simulink model "bh_6dof_NEWTON_vs_LAGRANGE"  (R2020b)
settings: Solver=ode23t  StartTime=0.0  StopTime=200  FixedStep=0.001  RelTol=1e-5  EnableMultiTasking=on
undefined symbols (not defined in the file or in its folder): P_elec, P_mot, P_one_prop, P_rot, P_veh, P_veh_no_props, sigbuilder_block
libraries: bh_6dof_LIBRARY x45, simulink_extras x37, pid_lib x24, simulink x6
(part 5 of 5)

== system bh_6dof_NEWTON_vs_LAGRANGE/PLANT VEHICLE_SYS1/bh_6DOF (Euler Angles, Lagrangian, Multi_body)/integrate/create_st_BUS ==
  e : Inport
  x : Inport  Port=2
  e_dot : Inport  Port=3
  x_dot : Inport  Port=4
  Bus Creator : BusCreator  Inputs=4
  Bus Creator1 : BusCreator  Inputs=6
  Bus Creator2 : BusCreator  Inputs=6
  Demux{,1..3} (4 alike) : Demux  Outputs=3
  Mux : Mux  Inputs=2
  Mux1 : Mux  Inputs=2
  Reshape1 : Reshape  OutputDimensionality=Column vector (2-D)
  Reshape8 : Reshape  OutputDimensionality=Column vector (2-D)
  state_BUS : Outport  VectorParamsAs1DForOutWhenUnconnected=off
  wires:
  e/1 -> Mux/1, [e]
  x/1 -> Mux/2, [x]
  e_dot/1 -> Mux1/1, [eD]
  x_dot/1 -> Mux1/2, [xD]
  Mux1/1 -> Reshape1/1
  Mux/1 -> Reshape8/1
  Reshape1/1 -> Bus Creator/2  "vel_col"
  Reshape8/1 -> Bus Creator/1  "pos_col"
  Bus Creator1/1 -> Bus Creator/3  "Pos_list"
  Demux/1 -> Bus Creator1/1  "Phi"
  Demux/2 -> Bus Creator1/2  "Theta"
  Demux/3 -> Bus Creator1/3  "Psi"
  Demux1/2 -> Bus Creator1/5  "Y"
  Demux1/3 -> Bus Creator1/6  "Z"
  Demux1/1 -> Bus Creator1/4  "X"
  [e] -> Demux/1
  [x] -> Demux1/1
  Bus Creator2/1 -> Bus Creator/4  "Vel_list"
  Demux2/1 -> Bus Creator2/1  "Phi_D"
  Demux2/2 -> Bus Creator2/2  "Theta_D"
  Demux2/3 -> Bus Creator2/3  "Psi_D"
  Demux3/1 -> Bus Creator2/4  "X_D"
  Demux3/2 -> Bus Creator2/5  "Y_D"
  Demux3/3 -> Bus Creator2/6  "Z_D"
  [eD] -> Demux2/1
  [xD] -> Demux3/1
  Bus Creator/1 -> state_BUS/1

== matlab function bh_6dof_NEWTON_vs_LAGRANGE/PLANT VEHICLE_SYS1/bh_6DOF (Euler Angles, Lagrangian, Multi_body)/MATLAB Function1 ==
  data: I input; Ixx output; Ixy output; Ixz output; Iyy output; Iyz output; Izz output
function [Ixx, Ixy, Ixz, Iyy, Iyz, Izz] = fcn(I)

Ixx = I(1,1); 
Ixy = I(1,2); 
Ixz = I(1,3); 
Iyy = I(2,2); 
Iyz = I(2,3); 
Izz = I(3,3);

end

== matlab function bh_6dof_NEWTON_vs_LAGRANGE/PLANT VEHICLE_SYS1/bh_6DOF (Euler Angles, Lagrangian, Multi_body)/MATLAB Function ==
  data: I input; Ixx output; Ixy output; Ixz output; Iyy output; Iyz output; Izz output
function [Ixx, Ixy, Ixz, Iyy, Iyz, Izz] = fcn(I)

Ixx = I(1,1); 
Ixy = I(1,2); 
Ixz = I(1,3); 
Iyy = I(2,2); 
Iyz = I(2,3); 
Izz = I(3,3);

end

== matlab function bh_6dof_NEWTON_vs_LAGRANGE/PLANT VEHICLE_SYS1/bh_6DOF (Euler Angles, Lagrangian, Multi_body)/Vg_to_Vb/bRg1 ==
  data: phi input; bRg output; theta input; psi input
function bRg = bRg(phi,theta,psi)
%#codegen

%    This function was generated by the Symbolic Math Toolbox version 7.2.
%    28-Aug-2017 09:46:25

bRg = reshape([cos(phi).*cos(theta),-cos(psi).*sin(phi)+cos(phi).*sin(psi).*sin(theta),sin(phi).*sin(psi)+cos(phi).*cos(psi).*sin(theta),cos(theta).*sin(phi),cos(phi).*cos(psi)+sin(phi).*sin(psi).*sin(theta),-cos(phi).*sin(psi)+cos(psi).*sin(phi).*sin(theta),-sin(theta),cos(theta).*sin(psi),cos(psi).*cos(theta)],[3,3]);

== matlab function bh_6dof_NEWTON_vs_LAGRANGE/PLANT VEHICLE_SYS1/bh_6DOF (Euler Angles, Lagrangian, Multi_body)/bRg ==
  data: phi input; bRg output; theta input; psi input
function bRg = bRg(phi,theta,psi)
%#codegen

%    This function was generated by the Symbolic Math Toolbox version 7.2.
%    28-Aug-2017 08:55:21

bRg = reshape([cos(phi).*cos(theta),-cos(psi).*sin(phi)+cos(phi).*sin(psi).*sin(theta),sin(phi).*sin(psi)+cos(phi).*cos(psi).*sin(theta),cos(theta).*sin(phi),cos(phi).*cos(psi)+sin(phi).*sin(psi).*sin(theta),-cos(phi).*sin(psi)+cos(psi).*sin(phi).*sin(theta),-sin(theta),cos(theta).*sin(psi),cos(psi).*cos(theta)],[3,3]);

== matlab function bh_6dof_NEWTON_vs_LAGRANGE/PLANT VEHICLE_SYS1/bh_6DOF (Euler Angles, Lagrangian, Multi_body)/MCKGQ1 ==
  data: I_xx input; M output; I_xy input; I_xz input; I_yy input; I_yz input; I_zz input; Iprop_xx input; Iprop_xy input; Iprop_xz input; Iprop_yy input; Iprop_yz input; Iprop_zz input; Mbz_1 input; Mbz_2 input; Mbz_3 input; Mbz_4 input; THE_Phi input; THE_Psi input; THE_Phi_D input; THE_Psi_D input; THE_Theta input; THE_Theta_D input; Tbz_1 input; Tbz_2 input; Tbz_3 input; Tbz_4 input; cg_to_mot_H input; cg_to_mot_L input; g input; m input; mprop input; wMOT_1 input; wMOT_2 input; wMOT_3 input; wMOT_4 input; C output; K output; G output; Q output
function [M,C,K,G,Q] = MCKGQ(I_xx,I_xy,I_xz,I_yy,I_yz,I_zz,Iprop_xx,Iprop_xy,Iprop_xz,Iprop_yy,Iprop_yz,Iprop_zz,Mbz_1,Mbz_2,Mbz_3,Mbz_4,THE_Phi,THE_Psi,THE_Phi_D,THE_Psi_D,THE_Theta,THE_Theta_D,Tbz_1,Tbz_2,Tbz_3,Tbz_4,cg_to_mot_H,cg_to_mot_L,g,m,mprop,wMOT_1,wMOT_2,wMOT_3,wMOT_4)
%#codegen

%    This function was generated by the Symbolic Math Toolbox version 7.2.
%    07-Sep-2017 08:25:18

M = reshape([I_xx+Iprop_xx.*4.0+cg_to_mot_H.^2.*mprop.*4.0+cg_to_mot_L.^2.*mprop.*2.0-I_xx.*cos(THE_Theta).^2+I_yy.*cos(THE_Theta).^2-Iprop_xx.*cos(THE_Theta).^2.*4.0+Iprop_yy.*cos(THE_Theta).^2.*4.0-I_yy.*cos(THE_Psi).^2.*cos(THE_Theta).^2+I_zz.*cos(THE_Psi).^2.*cos(THE_Theta).^2-Iprop_yy.*cos(THE_Psi).^2.*cos(THE_Theta).^2.*4.0+Iprop_zz.*cos(THE_Psi).^2.*cos(THE_Theta).^2.*4.0+I_yz.*cos(THE_Psi).*cos(THE_Theta).^2.*sin(THE_Psi).*2.0+Iprop_yz.*cos(THE_Psi).*cos(THE_Theta).^2.*sin(THE_Psi).*8.0-cg_to_mot_H.^2.*mprop.*cos(THE_Psi).^2.*cos(THE_Theta).^2.*4.0+cg_to_mot_L.^2.*mprop.*cos(THE_Psi).^2.*cos(THE_Theta).^2.*2.0-I_xz.*cos(THE_Psi).*cos(THE_Theta).*sin(THE_Theta).*2.0-Iprop_xz.*cos(THE_Psi).*cos(THE_Theta).*sin(THE_Theta).*8.0-I_xy.*cos(THE_Theta).*sin(THE_Psi).*sin(THE_Theta).*2.0-Iprop_xy.*cos(THE_Theta).*sin(THE_Psi).*sin(THE_Theta).*8.0,-I_yz.*cos(THE_Theta)-Iprop_yz.*cos(THE_Theta).*4.0-I_xy.*cos(THE_Psi).*sin(THE_Theta)-Iprop_xy.*cos(THE_Psi).*sin(THE_Theta).*4.0+I_xz.*sin(THE_Psi).*sin(THE_Theta)+Iprop_xz.*sin(THE_Psi).*sin(THE_Theta).*4.0+I_yz.*cos(THE_Psi).^2.*cos(THE_Theta).*2.0+Iprop_yz.*cos(THE_Psi).^2.*cos(THE_Theta).*8.0+I_yy.*cos(THE_Psi).*cos(THE_Theta).*sin(THE_Psi)-I_zz.*cos(THE_Psi).*cos(THE_Theta).*sin(THE_Psi)+Iprop_yy.*cos(THE_Psi).*cos(THE_Theta).*sin(THE_Psi).*4.0-Iprop_zz.*cos(THE_Psi).*cos(THE_Theta).*sin(THE_Psi).*4.0+cg_to_mot_H.^2.*mprop.*cos(THE_Psi).*cos(THE_Theta).*sin(THE_Psi).*4.0-cg_to_mot_L.^2.*mprop.*cos(THE_Psi).*cos(THE_Theta).*sin(THE_Psi).*2.0,-I_xx.*sin(THE_Theta)-Iprop_xx.*sin(THE_Theta).*4.0+I_xz.*cos(THE_Psi).*cos(THE_Theta)+Iprop_xz.*cos(THE_Psi).*cos(THE_Theta).*4.0+I_xy.*cos(THE_Theta).*sin(THE_Psi)+Iprop_xy.*cos(THE_Theta).*sin(THE_Psi).*4.0-cg_to_mot_H.^2.*mprop.*sin(THE_Theta).*4.0-cg_to_mot_L.^2.*mprop.*sin(THE_Theta).*2.0,cg_to_mot_H.*mprop.*(cos(THE_Phi).*sin(THE_Psi)-cos(THE_Psi).*sin(THE_Phi).*sin(THE_Theta)).*4.0,cg_to_mot_H.*mprop.*(sin(THE_Phi).*sin(THE_Psi)+cos(THE_Phi).*cos(THE_Psi).*sin(THE_Theta)).*4.0,0.0,-I_yz.*cos(THE_Theta)-Iprop_yz.*cos(THE_Theta).*4.0-I_xy.*cos(THE_Psi).*sin(THE_Theta)-Iprop_xy.*cos(THE_Psi).*sin(THE_Theta).*4.0+I_xz.*sin(THE_Psi).*sin(THE_Theta)+Iprop_xz.*sin(THE_Psi).*sin(THE_Theta).*4.0+I_yz.*cos(THE_Psi).^2.*cos(THE_Theta).*2.0+Iprop_yz.*cos(THE_Psi).^2.*cos(THE_Theta).*8.0+I_yy.*cos(THE_Psi).*cos(THE_Theta).*sin(THE_Psi)-I_zz.*cos(THE_Psi).*cos(THE_Theta).*sin(THE_Psi)+Iprop_yy.*cos(THE_Psi).*cos(THE_Theta).*sin(THE_Psi).*4.0-Iprop_zz.*cos(THE_Psi).*cos(THE_Theta).*sin(THE_Psi).*4.0+cg_to_mot_H.^2.*mprop.*cos(THE_Psi).*cos(THE_Theta).*sin(THE_Psi).*4.0-cg_to_mot_L.^2.*mprop.*cos(THE_Psi).*cos(THE_Theta).*sin(THE_Psi).*2.0,I_zz+Iprop_zz.*4.0+cg_to_mot_L.^2.*mprop.*4.0+I_yy.*cos(THE_Psi).^2-I_zz.*cos(THE_Psi).^2+Iprop_yy.*cos(THE_Psi).^2.*4.0-Iprop_zz.*cos(THE_Psi).^2.*4.0-I_yz.*sin(THE_Psi.*2.0)-Iprop_yz.*sin(THE_Psi.*2.0).*4.0+cg_to_mot_H.^2.*mprop.*cos(THE_Psi).^2.*4.0-cg_to_mot_L.^2.*mprop.*cos(THE_Psi).^2.*2.0,I_xy.*cos(THE_Psi)+Iprop_xy.*cos(THE_Psi).*4.0-I_xz.*sin(THE_Psi)-Iprop_xz.*sin(THE_Psi).*4.0,cg_to_mot_H.*mprop.*cos(THE_Phi).*cos(THE_Psi).*cos(THE_Theta).*4.0,cg_to_mot_H.*mprop.*cos(THE_Psi).*cos(THE_Theta).*sin(THE_Phi).*4.0,cg_to_mot_H.*mprop.*cos(THE_Psi).*sin(THE_Theta).*-4.0,-I_xx.*sin(THE_Theta)-Iprop_xx.*sin(THE_Theta).*4.0+I_xz.*cos(THE_Psi).*cos(THE_Theta)+Iprop_xz.*cos(THE_Psi).*cos(THE_Theta).*4.0+I_xy.*cos(THE_Theta).*sin(THE_Psi)+Iprop_xy.*cos(THE_Theta).*sin(THE_Psi).*4.0-cg_to_mot_H.^2.*mprop.*sin(THE_Theta).*4.0-cg_to_mot_L.^2.*mprop.*sin(THE_Theta).*2.0,I_xy.*cos(THE_Psi)+Iprop_xy.*cos(THE_Psi).*4.0-I_xz.*sin(THE_Psi)-Iprop_xz.*sin(THE_Psi).*4.0,I_xx+Iprop_xx.*4.0+cg_to_mot_H.^2.*mprop.*4.0+cg_to_mot_L.^2.*mprop.*2.0,cg_to_mot_H.*mprop.*(cos(THE_Psi).*sin(THE_Phi)-cos(THE_Phi).*sin(THE_Psi).*sin(THE_Theta)).*4.0,cg_to_mot_H.*mprop.*(cos(THE_Phi).*cos(THE_Psi)+sin(THE_Phi).*sin(THE_Psi).*sin(THE_Theta)).*-4.0,cg_to_mot_H.*mprop.*cos(THE_Theta).*sin(THE_Psi).*-4.0,cg_to_mot_H.*mprop.*(cos(THE_Phi).*sin(THE_Psi)-cos(THE_Psi).*sin(THE_Phi).*sin(THE_Theta)).*4.0,cg_to_mot_H.*mprop.*cos(THE_Phi).*cos(THE_Psi).*cos(THE_Theta).*4.0,cg_to_mot_H.*mprop.*(cos(THE_Psi).*sin(THE_Phi)-cos(THE_Phi).*sin(THE_Psi).*sin(THE_Theta)).*4.0,m+mprop.*4.0,0.0,0.0,cg_to_mot_H.*mprop.*(sin(THE_Phi).*sin(THE_Psi)+cos(THE_Phi).*cos(THE_Psi).*sin(THE_Theta)).*4.0,cg_to_mot_H.*mprop.*cos(THE_Psi).*cos(THE_Theta).*sin(THE_Phi).*4.0,cg_to_mot_H.*mprop.*(cos(THE_Phi).*cos(THE_Psi)+sin(THE_Phi).*sin(THE_Psi).*sin(THE_Theta)).*-4.0,0.0,m+mprop.*4.0,0.0,0.0,cg_to_mot_H.*mprop.*cos(THE_Psi).*sin(THE_Theta).*-4.0,cg_to_mot_H.*mprop.*cos(THE_Theta).*sin(THE_Psi).*-4.0,0.0,0.0,m+mprop.*4.0],[6,6]);
if nargout > 1
    C = reshape([I_yz.*THE_Psi_D.*cos(THE_Theta).^2.*-2.0-Iprop_yz.*THE_Psi_D.*cos(THE_Theta).^2.*8.0+I_xx.*THE_Theta_D.*sin(THE_Theta.*2.0)-I_yy.*THE_Theta_D.*sin(THE_Theta.*2.0)+Iprop_xx.*THE_Theta_D.*sin(THE_Theta.*2.0).*4.0-Iprop_yy.*THE_Theta_D.*sin(THE_Theta.*2.0).*4.0+I_xz.*THE_Theta_D.*cos(THE_Psi).*2.0+Iprop_xz.*THE_Theta_D.*cos(THE_Psi).*8.0+I_xy.*THE_Theta_D.*sin(THE_Psi).*2.0+Iprop_xy.*THE_Theta_D.*sin(THE_Psi).*8.0+I_yz.*THE_Psi_D.*cos(THE_Psi).^2.*cos(THE_Theta).^2.*4.0+Iprop_yz.*THE_Psi_D.*cos(THE_Psi).^2.*cos(THE_Theta).^2.*1.6e1-I_xz.*THE_Theta_D.*cos(THE_Psi).*cos(THE_Theta).^2.*4.0-Iprop_xz.*THE_Theta_D.*cos(THE_Psi).*cos(THE_Theta).^2.*1.6e1-I_xy.*THE_Theta_D.*cos(THE_Theta).^2.*sin(THE_Psi).*4.0-Iprop_xy.*THE_Theta_D.*cos(THE_Theta).^2.*sin(THE_Psi).*1.6e1-I_xy.*THE_Psi_D.*cos(THE_Psi).*cos(THE_Theta).*sin(THE_Theta).*2.0-Iprop_xy.*THE_Psi_D.*cos(THE_Psi).*cos(THE_Theta).*sin(THE_Theta).*8.0+I_xz.*THE_Psi_D.*cos(THE_Theta).*sin(THE_Psi).*sin(THE_Theta).*2.0+Iprop_xz.*THE_Psi_D.*cos(THE_Theta).*sin(THE_Psi).*sin(THE_Theta).*8.0+I_yy.*THE_Psi_D.*cos(THE_Psi).*cos(THE_Theta).^2.*sin(THE_Psi).*2.0-I_zz.*THE_Psi_D.*cos(THE_Psi).*cos(THE_Theta).^2.*sin(THE_Psi).*2.0+I_yy.*THE_Theta_D.*cos(THE_Psi).^2.*cos(THE_Theta).*sin(THE_Theta).*2.0-I_zz.*THE_Theta_D.*cos(THE_Psi).^2.*cos(THE_Theta).*sin(THE_Theta).*2.0+Iprop_yy.*THE_Psi_D.*cos(THE_Psi).*cos(THE_Theta).^2.*sin(THE_Psi).*8.0-Iprop_zz.*THE_Psi_D.*cos(THE_Psi).*cos(THE_Theta).^2.*sin(THE_Psi).*8.0+Iprop_yy.*THE_Theta_D.*cos(THE_Psi).^2.*cos(THE_Theta).*sin(THE_Theta).*8.0-Iprop_zz.*THE_Theta_D.*cos(THE_Psi).^2.*cos(THE_Theta).*sin(THE_Theta).*8.0+THE_Psi_D.*cg_to_mot_H.^2.*mprop.*cos(THE_Psi).*cos(THE_Theta).^2.*sin(THE_Psi).*8.0-THE_Psi_D.*cg_to_mot_L.^2.*mprop.*cos(THE_Psi).*cos(THE_Theta).^2.*sin(THE_Psi).*4.0+THE_Theta_D.*cg_to_mot_H.^2.*mprop.*cos(THE_Psi).^2.*cos(THE_Theta).*sin(THE_Theta).*8.0-THE_Theta_D.*cg_to_mot_L.^2.*mprop.*cos(THE_Psi).^2.*cos(THE_Theta).*sin(THE_Theta).*4.0-I_yz.*THE_Theta_D.*cos(THE_Psi).*cos(THE_Theta).*sin(THE_Psi).*sin(THE_Theta).*4.0-Iprop_yz.*THE_Theta_D.*cos(THE_Psi).*cos(THE_Theta).*sin(THE_Psi).*sin(THE_Theta).*1.6e1,I_xx.*THE_Phi_D.*sin(THE_Theta.*2.0).*(-1.0./2.0)+I_yy.*THE_Phi_D.*sin(THE_Theta.*2.0).*(1.0./2.0)-Iprop_xx.*THE_Phi_D.*sin(THE_Theta.*2.0).*2.0+Iprop_yy.*THE_Phi_D.*sin(THE_Theta.*2.0).*2.0-I_xz.*THE_Phi_D.*cos(THE_Psi)+I_xx.*THE_Psi_D.*cos(THE_Theta)-I_yy.*THE_Psi_D.*cos(THE_Theta)+I_zz.*THE_Psi_D.*cos(THE_Theta)-Iprop_xz.*THE_Phi_D.*cos(THE_Psi).*4.0+Iprop_xx.*THE_Psi_D.*cos(THE_Theta).*4.0-Iprop_yy.*THE_Psi_D.*cos(THE_Theta).*4.0+Iprop_zz.*THE_Psi_D.*cos(THE_Theta).*4.0-I_xy.*THE_Phi_D.*sin(THE_Psi)-Iprop_xy.*THE_Phi_D.*sin(THE_Psi).*4.0+Iprop_xz.*wMOT_1.*cos(THE_Theta)+Iprop_xz.*wMOT_2.*cos(THE_Theta)+Iprop_xz.*wMOT_3.*cos(THE_Theta)+Iprop_xz.*wMOT_4.*cos(THE_Theta)+I_xz.*THE_Psi_D.*cos(THE_Psi).*sin(THE_Theta).*2.0+Iprop_xz.*THE_Psi_D.*cos(THE_Psi).*sin(THE_Theta).*8.0+I_xy.*THE_Psi_D.*sin(THE_Psi).*sin(THE_Theta).*2.0+Iprop_xy.*THE_Psi_D.*sin(THE_Psi).*sin(THE_Theta).*8.0+THE_Psi_D.*cg_to_mot_L.^2.*mprop.*cos(THE_Theta).*4.0+Iprop_zz.*wMOT_1.*cos(THE_Psi).*sin(THE_Theta)+Iprop_zz.*wMOT_2.*cos(THE_Psi).*sin(THE_Theta)+Iprop_zz.*wMOT_3.*cos(THE_Psi).*sin(THE_Theta)+Iprop_zz.*wMOT_4.*cos(THE_Psi).*sin(THE_Theta)+Iprop_yz.*wMOT_1.*sin(THE_Psi).*sin(THE_Theta)+Iprop_yz.*wMOT_2.*sin(THE_Psi).*sin(THE_Theta)+Iprop_yz.*wMOT_3.*sin(THE_Psi).*sin(THE_Theta)+Iprop_yz.*wMOT_4.*sin(THE_Psi).*sin(THE_Theta)+I_xz.*THE_Phi_D.*cos(THE_Psi).*cos(THE_Theta).^2.*2.0+I_yy.*THE_Psi_D.*cos(THE_Psi).^2.*cos(THE_Theta).*2.0-I_zz.*THE_Psi_D.*cos(THE_Psi).^2.*cos(THE_Theta).*2.0+Iprop_xz.*THE_Phi_D.*cos(THE_Psi).*cos(THE_Theta).^2.*8.0+Iprop_yy.*THE_Psi_D.*cos(THE_Psi).^2.*cos(THE_Theta).*8.0-Iprop_zz.*THE_Psi_D.*cos(THE_Psi).^2.*cos(THE_Theta).*8.0+I_xy.*THE_Phi_D.*cos(THE_Theta).^2.*sin(THE_Psi).*2.0+Iprop_xy.*THE_Phi_D.*cos(THE_Theta).^2.*sin(THE_Psi).*8.0-I_yz.*THE_Psi_D.*cos(THE_Psi).*cos(THE_Theta).*sin(THE_Psi).*4.0-Iprop_yz.*THE_Psi_D.*cos(THE_Psi).*cos(THE_Theta).*sin(THE_Psi).*1.6e1-I_yy.*THE_Phi_D.*cos(THE_Psi).^2.*cos(THE_Theta).*sin(THE_Theta)+I_zz.*THE_Phi_D.*cos(THE_Psi).^2.*cos(THE_Theta).*sin(THE_Theta)-Iprop_yy.*THE_Phi_D.*cos(THE_Psi).^2.*cos(THE_Theta).*sin(THE_Theta).*4.0+Iprop_zz.*THE_Phi_D.*cos(THE_Psi).^2.*cos(THE_Theta).*sin(THE_Theta).*4.0+THE_Psi_D.*cg_to_mot_H.^2.*mprop.*cos(THE_Psi).^2.*cos(THE_Theta).*8.0-THE_Psi_D.*cg_to_mot_L.^2.*mprop.*cos(THE_Psi).^2.*cos(THE_Theta).*4.0-THE_Phi_D.*cg_to_mot_H.^2.*mprop.*cos(THE_Psi).^2.*cos(THE_Theta).*sin(THE_Theta).*4.0+THE_Phi_D.*cg_to_mot_L.^2.*mprop.*cos(THE_Psi).^2.*cos(THE_Theta).*sin(THE_Theta).*2.0+I_yz.*THE_Phi_D.*cos(THE_Psi).*cos(THE_Theta).*sin(THE_Psi).*sin(THE_Theta).*2.0+Iprop_yz.*THE_Phi_D.*cos(THE_Psi).*cos(THE_Theta).*sin(THE_Psi).*sin(THE_Theta).*8.0,I_yz.*THE_Phi_D.*cos(THE_Theta).^2+Iprop_yz.*THE_Phi_D.*cos(THE_Theta).^2.*4.0-I_xx.*THE_Theta_D.*cos(THE_Theta)+I_yy.*THE_Theta_D.*cos(THE_Theta)-I_zz.*THE_Theta_D.*cos(THE_Theta)-Iprop_xx.*THE_Theta_D.*cos(THE_Theta).*4.0+Iprop_yy.*THE_Theta_D.*cos(THE_Theta).*4.0-Iprop_zz.*THE_Theta_D.*cos(THE_Theta).*4.0-I_yz.*THE_Phi_D.*cos(THE_Psi).^2.*cos(THE_Theta).^2.*2.0-Iprop_yz.*THE_Phi_D.*cos(THE_Psi).^2.*cos(THE_Theta).^2.*8.0-I_xz.*THE_Theta_D.*cos(THE_Psi).*sin(THE_Theta).*2.0-Iprop_xz.*THE_Theta_D.*cos(THE_Psi).*sin(THE_Theta).*8.0-I_xy.*THE_Theta_D.*sin(THE_Psi).*sin(THE_Theta).*2.0-Iprop_xy.*THE_Theta_D.*sin(THE_Psi).*sin(THE_Theta).*8.0-Iprop_yz.*wMOT_1.*cos(THE_Psi).*cos(THE_Theta)-Iprop_yz.*wMOT_2.*cos(THE_Psi).*cos(THE_Theta)-Iprop_yz.*wMOT_3.*cos(THE_Psi).*cos(THE_Theta)-Iprop_yz.*wMOT_4.*cos(THE_Psi).*cos(THE_Theta)-THE_Theta_D.*cg_to_mot_L.^2.*mprop.*cos(THE_Theta).*4.0+Iprop_zz.*wMOT_1.*cos(THE_Theta).*sin(THE_Psi)+Iprop_zz.*wMOT_2.*cos(THE_Theta).*sin(THE_Psi)+Iprop_zz.*wMOT_3.*cos(THE_Theta).*sin(THE_Psi)+Iprop_zz.*wMOT_4.*cos(THE_Theta).*sin(THE_Psi)-I_yy.*THE_Theta_D.*cos(THE_Psi).^2.*cos(THE_Theta).*2.0+I_zz.*THE_Theta_D.*cos(THE_Psi).^2.*cos(THE_Theta).*2.0-Iprop_yy.*THE_Theta_D.*cos(THE_Psi).^2.*cos(THE_Theta).*8.0+Iprop_zz.*THE_Theta_D.*cos(THE_Psi).^2.*cos(THE_Theta).*8.0+I_xy.*THE_Phi_D.*cos(THE_Psi).*cos(THE_Theta).*sin(THE_Theta)+I_yz.*THE_Theta_D.*cos(THE_Psi).*cos(THE_Theta).*sin(THE_Psi).*4.0+Iprop_xy.*THE_Phi_D.*cos(THE_Psi).*cos(THE_Theta).*sin(THE_Theta).*4.0+Iprop_yz.*THE_Theta_D.*cos(THE_Psi).*cos(THE_Theta).*sin(THE_Psi).*1.6e1-I_xz.*THE_Phi_D.*cos(THE_Theta).*sin(THE_Psi).*sin(THE_Theta)-Iprop_xz.*THE_Phi_D.*cos(THE_Theta).*sin(THE_Psi).*sin(THE_Theta).*4.0-I_yy.*THE_Phi_D.*cos(THE_Psi).*cos(THE_Theta).^2.*sin(THE_Psi)+I_zz.*THE_Phi_D.*cos(THE_Psi).*cos(THE_Theta).^2.*sin(THE_Psi)-Iprop_yy.*THE_Phi_D.*cos(THE_Psi).*cos(THE_Theta).^2.*sin(THE_Psi).*4.0+Iprop_zz.*THE_Phi_D.*cos(THE_Psi).*cos(THE_Theta).^2.*sin(THE_Psi).*4.0-THE_Theta_D.*cg_to_mot_H.^2.*mprop.*cos(THE_Psi).^2.*cos(THE_Theta).*8.0+THE_Theta_D.*cg_to_mot_L.^2.*mprop.*cos(THE_Psi).^2.*cos(THE_Theta).*4.0-THE_Phi_D.*cg_to_mot_H.^2.*mprop.*cos(THE_Psi).*cos(THE_Theta).^2.*sin(THE_Psi).*4.0+THE_Phi_D.*cg_to_mot_L.^2.*mprop.*cos(THE_Psi).*cos(THE_Theta).^2.*sin(THE_Psi).*2.0,cg_to_mot_H.*mprop.*(THE_Psi_D.*cos(THE_Phi).*cos(THE_Psi).*-2.0+THE_Phi_D.*sin(THE_Phi).*sin(THE_Psi)-THE_Psi_D.*sin(THE_Phi).*sin(THE_Psi).*sin(THE_Theta).*2.0+THE_Phi_D.*cos(THE_Phi).*cos(THE_Psi).*sin(THE_Theta)+THE_Theta_D.*cos(THE_Psi).*cos(THE_Theta).*sin(THE_Phi).*2.0).*-4.0,cg_to_mot_H.*mprop.*(THE_Phi_D.*cos(THE_Phi).*sin(THE_Psi)+THE_Psi_D.*cos(THE_Psi).*sin(THE_Phi).*2.0+THE_Theta_D.*cos(THE_Phi).*cos(THE_Psi).*cos(THE_Theta).*2.0-THE_Phi_D.*cos(THE_Psi).*sin(THE_Phi).*sin(THE_Theta)-THE_Psi_D.*cos(THE_Phi).*sin(THE_Psi).*sin(THE_Theta).*2.0).*4.0,0.0,-I_xx.*THE_Psi_D.*cos(THE_Theta)-I_yy.*THE_Psi_D.*cos(THE_Theta)+I_zz.*THE_Psi_D.*cos(THE_Theta)-Iprop_xx.*THE_Psi_D.*cos(THE_Theta).*4.0-Iprop_yy.*THE_Psi_D.*cos(THE_Theta).*4.0+Iprop_zz.*THE_Psi_D.*cos(THE_Theta).*4.0+I_yz.*THE_Theta_D.*sin(THE_Theta)+Iprop_yz.*THE_Theta_D.*sin(THE_Theta).*4.0-Iprop_xz.*wMOT_1.*cos(THE_Theta)-Iprop_xz.*wMOT_2.*cos(THE_Theta)-Iprop_xz.*wMOT_3.*cos(THE_Theta)-Iprop_xz.*wMOT_4.*cos(THE_Theta)-I_xy.*THE_Theta_D.*cos(THE_Psi).*cos(THE_Theta)-Iprop_xy.*THE_Theta_D.*cos(THE_Psi).*cos(THE_Theta).*4.0+I_xz.*THE_Theta_D.*cos(THE_Theta).*sin(THE_Psi)+Iprop_xz.*THE_Theta_D.*cos(THE_Theta).*sin(THE_Psi).*4.0-THE_Psi_D.*cg_to_mot_H.^2.*mprop.*cos(THE_Theta).*8.0-Iprop_zz.*wMOT_1.*cos(THE_Psi).*sin(THE_Theta)-Iprop_zz.*wMOT_2.*cos(THE_Psi).*sin(THE_Theta)-Iprop_zz.*wMOT_3.*cos(THE_Psi).*sin(THE_Theta)-Iprop_zz.*wMOT_4.*cos(THE_Psi).*sin(THE_Theta)-Iprop_yz.*wMOT_1.*sin(THE_Psi).*sin(THE_Theta)-Iprop_yz.*wMOT_2.*sin(THE_Psi).*sin(THE_Theta)-Iprop_yz.*wMOT_3.*sin(THE_Psi).*sin(THE_Theta)-Iprop_yz.*wMOT_4.*sin(THE_Psi).*sin(THE_Theta)+I_yy.*THE_Psi_D.*cos(THE_Psi).^2.*cos(THE_Theta).*2.0-I_zz.*THE_Psi_D.*cos(THE_Psi).^2.*cos(THE_Theta).*2.0+Iprop_yy.*THE_Psi_D.*cos(THE_Psi).^2.*cos(THE_Theta).*8.0-Iprop_zz.*THE_Psi_D.*cos(THE_Psi).^2.*cos(THE_Theta).*8.0-I_yz.*THE_Theta_D.*cos(THE_Psi).^2.*sin(THE_Theta).*2.0-Iprop_yz.*THE_Theta_D.*cos(THE_Psi).^2.*sin(THE_Theta).*8.0-I_yz.*THE_Psi_D.*cos(THE_Psi).*cos(THE_Theta).*sin(THE_Psi).*4.0-Iprop_yz.*THE_Psi_D.*cos(THE_Psi).*cos(THE_Theta).*sin(THE_Psi).*1.6e1-I_yy.*THE_Theta_D.*cos(THE_Psi).*sin(THE_Psi).*sin(THE_Theta)+I_zz.*THE_Theta_D.*cos(THE_Psi).*sin(THE_Psi).*sin(THE_Theta)-Iprop_yy.*THE_Theta_D.*cos(THE_Psi).*sin(THE_Psi).*sin(THE_Theta).*4.0+Iprop_zz.*THE_Theta_D.*cos(THE_Psi).*sin(THE_Psi).*sin(THE_Theta).*4.0+THE_Psi_D.*cg_to_mot_H.^2.*mprop.*cos(THE_Psi).^2.*cos(THE_Theta).*8.0-THE_Psi_D.*cg_to_mot_L.^2.*mprop.*cos(THE_Psi).^2.*cos(THE_Theta).*4.0-THE_Theta_D.*cg_to_mot_H.^2.*mprop.*cos(THE_Psi).*sin(THE_Psi).*sin(THE_Theta).*4.0+THE_Theta_D.*cg_to_mot_L.^2.*mprop.*cos(THE_Psi).*sin(THE_Psi).*sin(THE_Theta).*2.0,-THE_Psi_D.*(I_yz.*cos(THE_Psi.*2.0).*2.0+Iprop_yz.*cos(THE_Psi.*2.0).*8.0+I_yy.*sin(THE_Psi.*2.0)-I_zz.*sin(THE_Psi.*2.0)+Iprop_yy.*sin(THE_Psi.*2.0).*4.0-Iprop_zz.*sin(THE_Psi.*2.0).*4.0+cg_to_mot_H.^2.*mprop.*sin(THE_Psi.*2.0).*4.0-cg_to_mot_L.^2.*mprop.*sin(THE_Psi.*2.0).*2.0),I_yz.*THE_Theta_D.*cos(THE_Psi.*2.0)+Iprop_yz.*THE_Theta_D.*cos(THE_Psi.*2.0).*4.0+I_yy.*THE_Theta_D.*sin(THE_Psi.*2.0).*(1.0./2.0)-I_zz.*THE_Theta_D.*sin(THE_Psi.*2.0).*(1.0./2.0)+Iprop_yy.*THE_Theta_D.*sin(THE_Psi.*2.0).*2.0-Iprop_zz.*THE_Theta_D.*sin(THE_Psi.*2.0).*2.0+Iprop_zz.*wMOT_1.*cos(THE_Psi)+Iprop_zz.*wMOT_2.*cos(THE_Psi)+Iprop_zz.*wMOT_3.*cos(THE_Psi)+Iprop_zz.*wMOT_4.*cos(THE_Psi)+Iprop_yz.*wMOT_1.*sin(THE_Psi)+Iprop_yz.*wMOT_2.*sin(THE_Psi)+Iprop_yz.*wMOT_3.*sin(THE_Psi)+Iprop_yz.*wMOT_4.*sin(THE_Psi)+THE_Theta_D.*cg_to_mot_H.^2.*mprop.*sin(THE_Psi.*2.0).*2.0-THE_Theta_D.*cg_to_mot_L.^2.*mprop.*sin(THE_Psi.*2.0),cg_to_mot_H.*mprop.*cos(THE_Phi).*(THE_Psi_D.*cos(THE_Theta).*sin(THE_Psi).*2.0+THE_Theta_D.*cos(THE_Psi).*sin(THE_Theta)).*-4.0,cg_to_mot_H.*mprop.*sin(THE_Phi).*(THE_Psi_D.*cos(THE_Theta).*sin(THE_Psi).*2.0+THE_Theta_D.*cos(THE_Psi).*sin(THE_Theta)).*-4.0,cg_to_mot_H.*mprop.*(THE_Theta_D.*cos(THE_Psi).*cos(THE_Theta)-THE_Psi_D.*sin(THE_Psi).*sin(THE_Theta).*2.0).*-4.0,cos(THE_Theta).*(I_xy.*THE_Psi_D.*cos(THE_Psi)+Iprop_xy.*THE_Psi_D.*cos(THE_Psi).*4.0-I_xz.*THE_Psi_D.*sin(THE_Psi)-Iprop_xz.*THE_Psi_D.*sin(THE_Psi).*4.0+Iprop_yz.*wMOT_1.*cos(THE_Psi)+Iprop_yz.*wMOT_2.*cos(THE_Psi)+Iprop_yz.*wMOT_3.*cos(THE_Psi)+Iprop_yz.*wMOT_4.*cos(THE_Psi)-Iprop_zz.*wMOT_1.*sin(THE_Psi)-Iprop_zz.*wMOT_2.*sin(THE_Psi)-Iprop_zz.*wMOT_3.*sin(THE_Psi)-Iprop_zz.*wMOT_4.*sin(THE_Psi)),-I_xz.*THE_Psi_D.*cos(THE_Psi)-Iprop_xz.*THE_Psi_D.*cos(THE_Psi).*4.0-I_xy.*THE_Psi_D.*sin(THE_Psi)-Iprop_xy.*THE_Psi_D.*sin(THE_Psi).*4.0-Iprop_zz.*wMOT_1.*cos(THE_Psi)-Iprop_zz.*wMOT_2.*cos(THE_Psi)-Iprop_zz.*wMOT_3.*cos(THE_Psi)-Iprop_zz.*wMOT_4.*cos(THE_Psi)-Iprop_yz.*wMOT_1.*sin(THE_Psi)-Iprop_yz.*wMOT_2.*sin(THE_Psi)-Iprop_yz.*wMOT_3.*sin(THE_Psi)-Iprop_yz.*wMOT_4.*sin(THE_Psi),0.0,THE_Psi_D.*cg_to_mot_H.*mprop.*(sin(THE_Phi).*sin(THE_Psi)+cos(THE_Phi).*cos(THE_Psi).*sin(THE_Theta)).*-4.0,THE_Psi_D.*cg_to_mot_H.*mprop.*(cos(THE_Phi).*sin(THE_Psi)-cos(THE_Psi).*sin(THE_Phi).*sin(THE_Theta)).*4.0,THE_Psi_D.*cg_to_mot_H.*mprop.*cos(THE_Psi).*cos(THE_Theta).*-4.0,0.0,0.0,0.0,0.0,0.0,0.0,0.0,0.0,0.0,0.0,0.0,0.0,0.0,0.0,0.0,0.0,0.0,0.0],[6,6]);
end
if nargout > 2
    K = reshape([0.0,0.0,0.0,0.0,0.0,0.0,0.0,0.0,0.0,0.0,0.0,0.0,0.0,0.0,0.0,0.0,0.0,0.0,0.0,0.0,0.0,0.0,0.0,0.0,0.0,0.0,0.0,0.0,0.0,0.0,0.0,0.0,0.0,0.0,0.0,0.0],[6,6]);
end
if nargout > 3
    G = [0.0;cg_to_mot_H.*g.*mprop.*cos(THE_Psi).*sin(THE_Theta).*-4.0;cg_to_mot_H.*g.*mprop.*cos(THE_Theta).*sin(THE_Psi).*-4.0;0.0;0.0;g.*(m+mprop.*4.0)];
end
if nargout > 4
    Q = [Mbz_1.*cos(THE_Psi).*cos(THE_Theta)+Mbz_2.*cos(THE_Psi).*cos(THE_Theta)+Mbz_3.*cos(THE_Psi).*cos(THE_Theta)+Mbz_4.*cos(THE_Psi).*cos(THE_Theta)-Tbz_2.*cg_to_mot_L.*sin(THE_Theta)+Tbz_4.*cg_to_mot_L.*sin(THE_Theta)-Tbz_1.*cg_to_mot_L.*cos(THE_Theta).*sin(THE_Psi)+Tbz_3.*cg_to_mot_L.*cos(THE_Theta).*sin(THE_Psi);-Mbz_1.*sin(THE_Psi)-Mbz_2.*sin(THE_Psi)-Mbz_3.*sin(THE_Psi)-Mbz_4.*sin(THE_Psi)-Tbz_1.*cg_to_mot_L.*cos(THE_Psi)+Tbz_3.*cg_to_mot_L.*cos(THE_Psi);cg_to_mot_L.*(Tbz_2-Tbz_4);(sin(THE_Phi).*sin(THE_Psi)+cos(THE_Phi).*cos(THE_Psi).*sin(THE_Theta)).*(Tbz_1+Tbz_2+Tbz_3+Tbz_4);-(cos(THE_Phi).*sin(THE_Psi)-cos(THE_Psi).*sin(THE_Phi).*sin(THE_Theta)).*(Tbz_1+Tbz_2+Tbz_3+Tbz_4);cos(THE_Psi).*cos(THE_Theta).*(Tbz_1+Tbz_2+Tbz_3+Tbz_4)];
end

== matlab function bh_6dof_NEWTON_vs_LAGRANGE/PLANT VEHICLE_SYS1/bh_6DOF (Euler Angles, Lagrangian, Multi_body)/integrate/bRg ==
  data: phi input; bRg output; theta input; psi input
function bRg = bRg(phi,theta,psi)
%#codegen

%    This function was generated by the Symbolic Math Toolbox version 7.2.
%    28-Aug-2017 10:05:16

bRg = reshape([cos(phi).*cos(theta),-cos(psi).*sin(phi)+cos(phi).*sin(psi).*sin(theta),sin(phi).*sin(psi)+cos(phi).*cos(psi).*sin(theta),cos(theta).*sin(phi),cos(phi).*cos(psi)+sin(phi).*sin(psi).*sin(theta),-cos(phi).*sin(psi)+cos(psi).*sin(phi).*sin(theta),-sin(theta),cos(theta).*sin(psi),cos(psi).*cos(theta)],[3,3]);

== matlab function bh_6dof_NEWTON_vs_LAGRANGE/PLANT VEHICLE_SYS1/bh_6DOF (Euler Angles, Lagrangian, Multi_body)/integrate/calc_eul_rates_from_w ==
  data: THE_Theta input; edot output; THE_Psi input; p input; q input; r input
function edot = calc_eul_rates_from_w(THE_Theta,THE_Psi,p,q,r)
%#codegen

%    This function was generated by the Symbolic Math Toolbox version 7.2.
%    28-Aug-2017 10:05:22

edot = [(r.*cos(THE_Psi)+q.*sin(THE_Psi))./cos(THE_Theta);q.*cos(THE_Psi)-r.*sin(THE_Psi);(p.*cos(THE_Theta)+r.*cos(THE_Psi).*sin(THE_Theta)+q.*sin(THE_Psi).*sin(THE_Theta))./cos(THE_Theta)];

== matlab function bh_6dof_NEWTON_vs_LAGRANGE/PLANT VEHICLE_SYS1/bh_6DOF (Euler Angles, Lagrangian, Multi_body)/solve_for_qDD/MATLAB Function ==
  data: M input; the_cond output
function the_cond = COND(M)
%#codegen

the_cond = cond(M);

end

== matlab function bh_6dof_NEWTON_vs_LAGRANGE/CONT_SYS W_MOT_CMDS1/w2toFM1 ==
  data: L input; Tbz_col output; Thrust_const input; Twist_const input; w2_col input; Mbz_col output; wM_col output
function [Tbz_col, Mbz_col, wM_col] = w2toFM(L, Thrust_const, Twist_const, w2_col)
%#codegen

    % simplify the variable names
    b = Thrust_const;
    k = Twist_const;

    % construct the co-efficient matrix:
    %  F_and_M = C * w^2
    
%     C = [     b,    b,    b,    b;
%               0,    b*L,  0,   -b*L;
%              -b*L,  0,    b*L,  0;
%              -k,    k,   -k,    k; ];

    Tbz_col = [ b; b; b; b ]  .*  w2_col;     
    Mbz_col = [-k; k;-k; k ]  .*  w2_col;          
    wM_col  = [ 1;-1; 1;-1 ]  .*  sqrt(w2_col); 
end

== matlab function bh_6dof_NEWTON_vs_LAGRANGE/CONT_SYS W_MOT_CMDS1/w2toFM2 ==
  data: L input; Thrust output; Thrust_const input; Twist_const input; w2_col input; TQ_roll_X output; TQ_pit_Y output; TQ_yaw_Z output
function [Thrust, TQ_roll_X, TQ_pit_Y, TQ_yaw_Z] = w2toFM(L, Thrust_const, Twist_const, w2_col)
%#codegen

    % simplify the variable names
    b = Thrust_const;
    k = Twist_const;

    % construct the co-efficient matrix:
    %  F_and_M = C * w^2
    
    C = [     b,    b,    b,    b;
              0,    b*L,  0,   -b*L;
             -b*L,  0,    b*L,  0;
             -k,    k,   -k,    k; ];

    % solve for the FM_col
    %   FM_col = [Thrust, TQ_roll_X, TQ_pit_Y, TQ_yaw_Z].' ;
    
    FM_col  =  C * w2_col;
    
    Thrust    =  FM_col(1);
    TQ_roll_X =  FM_col(2);
    TQ_pit_Y  =  FM_col(3);
    TQ_yaw_Z  =  FM_col(4);
    
end

== matlab function bh_6dof_NEWTON_vs_LAGRANGE/PLANT VEHICLE_SYS1/bh_6DOF (Euler Angles, Lagrangian, Multi_body)/calc_wb/calc_w_from_eul_rates ==
  data: THE_Theta input; wb output; THE_Psi input; THE_PhiD input; THE_ThetaD input; THE_PsiD input
function wb = calc_w_from_eul_rates(THE_Theta,THE_Psi,THE_PhiD,THE_ThetaD,THE_PsiD)
%#codegen

%    This function was generated by the Symbolic Math Toolbox version 7.2.
%    28-Aug-2017 10:05:21

wb = [THE_PsiD-THE_PhiD.*sin(THE_Theta);THE_ThetaD.*cos(THE_Psi)+THE_PhiD.*cos(THE_Theta).*sin(THE_Psi);-THE_ThetaD.*sin(THE_Psi)+THE_PhiD.*cos(THE_Psi).*cos(THE_Theta)];

== matlab function bh_6dof_NEWTON_vs_LAGRANGE/CONT_SYS Force_Moment_CMDS1/PITCH_and_ROLL_CONT/MATLAB Function ==
  data: Gr input size=[2 1]; Qr output size=[2 1]; ang input size=[1 1]
function Qr = fcn(Gr, ang)
%#codegen

    bRg = [  cos(ang),  sin(ang);
            -sin(ang),  cos(ang);
          ];  

    Qr = bRg * Gr;
end

== matlab function bh_6dof_NEWTON_vs_LAGRANGE/CONT_SYS W_MOT_CMDS/FM_to_w2 ==
  data: L input; w2_cmd output; Thrust_const input; Twist_const input; Thrust input; TQ_roll_X input; TQ_pit_Y input; TQ_yaw_Z input
function w2_cmd = FMtow2(L, Thrust_const, Twist_const, Thrust, TQ_roll_X, TQ_pit_Y, TQ_yaw_Z)
%#codegen

    % simplify the variable names
    b = Thrust_const;
    k = Twist_const;

    % construct the co-efficient matrix:
    %  F_and_M = C * w^2
    %
    % C = [     b,    b,    b,    b;
    %           0,    b*L,  0,   -b*L;
    %          -b*L,  0,    b*L,  0;
    %          -k,    k,   -k,    k; ];

    % used Symbolic toolbox to compute inv(C)
    C_inv = [
             1/(4*b),          0, -1/(2*L*b), -1/(4*k);
             1/(4*b),  1/(2*L*b),          0,  1/(4*k);
             1/(4*b),          0,  1/(2*L*b), -1/(4*k);
             1/(4*b), -1/(2*L*b),          0,  1/(4*k);
            ];
    % solve for the w^2 vec
    F_and_M_col = [Thrust, TQ_roll_X, TQ_pit_Y, TQ_yaw_Z].' ;

    w2_cmd = C_inv * F_and_M_col;
    
    tf_col = (w2_cmd >= 0);
   assert(all(w2_cmd), 'ERROR: some w2 are NEGATIVE !')
   %assert(false, 'ERROR: some w2 are NEGATIVE !')
end

== matlab function bh_6dof_NEWTON_vs_LAGRANGE/CONT_SYS W_MOT_CMDS/w2toFM ==
  data: L input; Thrust output; Thrust_const input; Twist_const input; w2_col input; TQ_roll_X output; TQ_pit_Y output; TQ_yaw_Z output
function [Thrust, TQ_roll_X, TQ_pit_Y, TQ_yaw_Z] = w2toFM(L, Thrust_const, Twist_const, w2_col)
%#codegen

    % simplify the variable names
    b = Thrust_const;
    k = Twist_const;

    % construct the co-efficient matrix:
    %  F_and_M = C * w^2
    
    C = [     b,    b,    b,    b;
              0,    b*L,  0,   -b*L;
             -b*L,  0,    b*L,  0;
             -k,    k,   -k,    k; ];

    % solve for the FM_col
    %   FM_col = [Thrust, TQ_roll_X, TQ_pit_Y, TQ_yaw_Z].' ;
    
    FM_col  =  C * w2_col;
    
    Thrust    =  FM_col(1);
    TQ_roll_X =  FM_col(2);
    TQ_pit_Y  =  FM_col(3);
    TQ_yaw_Z  =  FM_col(4);
    
end

== matlab function bh_6dof_NEWTON_vs_LAGRANGE/CONT_SYS Force_Moment_CMDS/PITCH_and_ROLL_CONT/MATLAB Function ==
  data: Gr input size=[2 1]; Qr output size=[2 1]; ang input size=[1 1]
function Qr = fcn(Gr, ang)
%#codegen

    bRg = [  cos(ang),  sin(ang);
            -sin(ang),  cos(ang);
          ];  

    Qr = bRg * Gr;
end

== matlab function bh_6dof_NEWTON_vs_LAGRANGE/CONT_SYS W_MOT_CMDS1/FM_to_w2 ==
  data: L input; w2_cmd output; Thrust_const input; Twist_const input; Thrust input; TQ_roll_X input; TQ_pit_Y input; TQ_yaw_Z input
function w2_cmd = FMtow2(L, Thrust_const, Twist_const, Thrust, TQ_roll_X, TQ_pit_Y, TQ_yaw_Z)
%#codegen

    % simplify the variable names
    b = Thrust_const;
    k = Twist_const;

    % construct the co-efficient matrix:
    %  F_and_M = C * w^2
    %
    % C = [     b,    b,    b,    b;
    %           0,    b*L,  0,   -b*L;
    %          -b*L,  0,    b*L,  0;
    %          -k,    k,   -k,    k; ];

    % used Symbolic toolbox to compute inv(C)
    C_inv = [
             1/(4*b),          0, -1/(2*L*b), -1/(4*k);
             1/(4*b),  1/(2*L*b),          0,  1/(4*k);
             1/(4*b),          0,  1/(2*L*b), -1/(4*k);
             1/(4*b), -1/(2*L*b),          0,  1/(4*k);
            ];
    % solve for the w^2 vec
    F_and_M_col = [Thrust, TQ_roll_X, TQ_pit_Y, TQ_yaw_Z].' ;

    w2_cmd = C_inv * F_and_M_col;
    
    tf_col = (w2_cmd >= 0);
   assert(all(w2_cmd), 'ERROR: some w2 are NEGATIVE !')
   %assert(false, 'ERROR: some w2 are NEGATIVE !')
end
